simulink subsystem "vehicle_sim"  (R2025b)
settings: Solver=VariableStepAuto  StartTime=0.0  StopTime=10.0  RelTol=1e-3
libraries: vehdynlibsteering x1, autolibshared x1
settings Model: Creator=jessi  LastModifiedBy=jessi

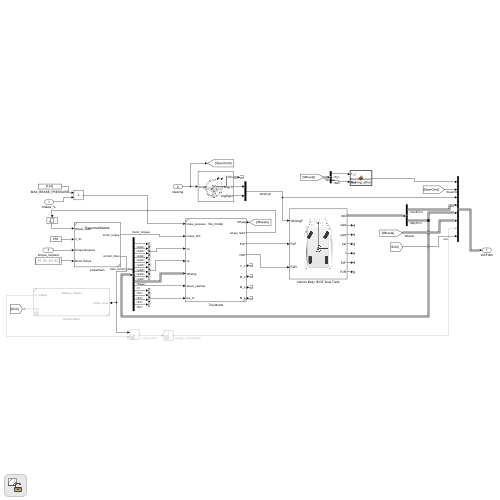
[thumbnail: Simulink's stored preview of the top-level diagram]
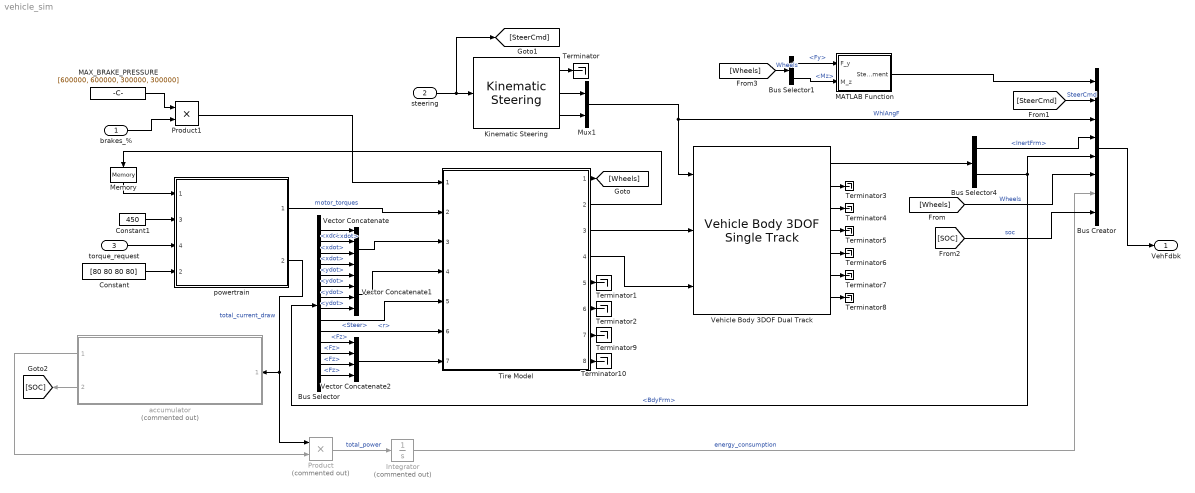
== system vehicle_sim ==
  brakes_% : Inport  PortDimensions=1
  steering : Inport  Port=2
  torque_request : Inport  Port=3  Unit=N*m  PortDimensions=4
  Bus Creator : BusCreator  Inputs=8
  Bus Selector : BusSelector  OutputSignals=FrntAxl.Lft.Vel.xdot,FrntAxl.Rght.Vel.xdot,RearAxl.Lft.Vel.xdot,RearAxl.Rght.Vel.xdot,FrntAxl.Lft.Vel.ydot,FrntAxl.Rght.Vel.ydot,RearAxl.Lft.Vel.ydot,RearAxl.Rght.Vel.ydot,FrntAxl.Steer,Cg.AngVel.r,Forces.Tires.FrntTires.Lft.Fz,Forces.Tires.FrntTires.Rght.Fz,Forces.Tires.RearTires.Lft.Fz,Forces.Tires.RearTires.Rght.Fz
  Bus Selector1 : BusSelector  OutputSignals=Fy,Mz
  Bus Selector4 : BusSelector  OutputSignals=InertFrm,BdyFrm
  Constant : Constant  Value=[80 80 80 80]
  Constant1 : Constant  Value=450
  Integrator : Integrator  Commented=on
  Kinematic Steering : vehdynlibsteering/Kinematic Steering  StrgType=Ackerman  StrgRatioType=Constant  Loc=Front  NrmlFctr=1  TrckWdth=1.1  WhlBase=1.550  Db=0  StrgRng=3*pi  StrgAngBpts="[-6.2832   -5.0265   -3.7699   -2.5133   -1.2566         0    1.2566    2.5133    3.7699    5.0265    6.2832]"  StrgRatioTbl=|  StrgRatio=10  PctAckIn=off  PctAck=100  PctAckTbl=ones(1,11)*100  StrgArmLngth=0.1  RckCsLngth=0.5  TieRodLngth=0.248  D=0.2  PnnRadius=0.00085818  PnnRadiusTbl="[0.0055    0.0055    0.0056    0.0057    0.0058    0.0057    0.0057    0.0057    0.0056    0.0055    0.0055]"  RodLngth=0.1  ParaArmLngth=0.9  aMode=2
      | [13.5000   13.3750   13.2500   13.1250   13.0000   13.0000   13.0000   13.1250   13.2500   13.3750   13.5000
      | ]
  MATLAB Function : MATLAB Function  TreatAsAtomicUnit=on
  MAX_BRAKE_PRESSURE : Constant  Value=[600000, 600000, 300000, 300000]
  Memory : Memory
  Mux1 : Mux  Inputs=2
  Product : Product  Commented=on
  Product1 : Product
  Terminator{,1..10} (11 alike) : Terminator
  Tire Model : Subsystem  ReferencedSubsystem=tire_model
  Vector Concatenate : Concatenate  NumInputs=4
  Vector Concatenate1 : Concatenate  NumInputs=4
  Vector Concatenate2 : Concatenate  NumInputs=4
  Vehicle Body 3DOF Dual Track : autolibshared/Vehicle Body 3DOF Single Track  trackMode=Dual  inputMode=External forces  frontSteerMode=on  rearSteerMode=off  windMode=off  muMode=off  extFMode=off  extMMode=off  htchFMode=off  htchMMode=off  extXo=off  extpsio=off  extxdoto=off  extro=off  extYo=off  extTamb=off  extydoto=off  aMode=2  NF=2  NR=2  m=252  a=0.803  b=0.747  h=0.20  dh=1  hh=0.2  X_o=0  xdot_o=0.1  CalphaMode=off  sigmaMode=on  d=0  hl=0  w=[0.775, 0.775]  Cy_f=12e3  Cy_r=11e3  sigma_f=.1  sigma_r=.1  alpha_f_brk=[-.1 .1]  Cy_f_data=[-9e3 9e3]  alpha_r_brk=[-.1 .1]  Cy_r_data=[-9e3 9e3]  Y_o=0  ydot_o=0  Izz=400  psi_o=0  r_o=0  Af=0.94  Cd=1.08  Cl=1.52  Cpm=.1  beta_w=[0 0.01:0.01:0.3]  Cs=[0:0.03:0.9]  Cym=[0 1e-6:0.01:0.3]  Pabs=101325  Tair=303  g=9.81  mu=1  xdot_tol=.01  Fznom=1961  Fxtire_sat=7e4  Fytire_sat=7e4  longOff=0  latOff=0  vertOff=0  wrapAng=off
      settings: LibrarySourceBlock=vehdynlibeom/Vehicle Body 3DOF Dual Track
  accumulator : Subsystem  Commented=on  ReferencedSubsystem=battery_model
      settings: PermitHierarchicalResolution=None
  powertrain : Subsystem  ReferencedSubsystem=PowertrainMatlab
      settings: PortSchema="{\"entries\":[{\"content\":{\"sides\":[{\"content\":{\"connectorIds\":[\"In1\",\"In3\",\"In4\",\"In2\"]},\"type\":\"ConnectorPlacement.EquallySpacedRectSide\",\"uuid\":\"bcaef28c-3728-4a2f-bdf4-b5e563d052c4\"},{\"content\":{\"connectorIds\":[\"Out1\",\"Out2\"],\"side\":\"RIGHT\"},\"type\":\"ConnectorPlacement.EquallySpacedRectSide\",\"uuid\":\"28426850-3a4f-491f-93a4-dadf03d879c7\"},{\"content\":{\"side\":\"TOP\"},\"type\":\"ConnectorPlacement.EquallySpacedRectSide\",\"uuid\":\"e3e154eb-71d0-41ee-9d2f-ecd68212e3aa\"}]},\"type\":\"ConnectorPlacement.EquallySpacedConnector\",\"uuid\":\"36c75ed7-43f2-403e-a237-5cc8486f527e\"}],\"packageUris\":[\"http://schema.mathworks.com/mf0/Connector/R2020b\"],\"version\":\"1.0\"}"
  VehFdbk : Outport
  wires:
  Bus Creator/1 -> VehFdbk/1
  Memory/1 -> powertrain/1
  Tire Model/8 -> Terminator10/1
  Tire Model/7 -> Terminator9/1
  Tire Model/6 -> Terminator2/1
  Tire Model/5 -> Terminator1/1
  brakes_%/1 -> Product1/2
  Bus Selector/3 -> Vector Concatenate/3  "<xdot>"
  Constant/1 -> powertrain/2
  Mux1/1 -> Vehicle Body 3DOF Dual Track/1, Bus Creator/3  "WhlAngF"
  Vehicle Body 3DOF Dual Track/5 -> Terminator6/1
  Bus Selector4/2 -> Bus Selector/1, Bus Creator/5  "<BdyFrm>"
  Bus Selector/7 -> Vector Concatenate1/3  "<ydot>"
  Bus Selector/13 -> Vector Concatenate2/3  "<Fz>"
  Bus Selector/11 -> Vector Concatenate2/1  "<Fz>"
  Bus Selector/5 -> Vector Concatenate1/1  "<ydot>"
  Vehicle Body 3DOF Dual Track/6 -> Terminator7/1
  Product/1 -> Integrator/1  "total_power"
  Bus Selector/1 -> Vector Concatenate/1  "<xdot>"
  Vehicle Body 3DOF Dual Track/3 -> Terminator4/1
  Bus Selector/6 -> Vector Concatenate1/2  "<ydot>"
  Kinematic Steering/1 -> Terminator/1
  Bus Selector/4 -> Vector Concatenate/4  "<xdot>"
  Vehicle Body 3DOF Dual Track/4 -> Terminator5/1
  Bus Selector/8 -> Vector Concatenate1/4  "<ydot>"
  accumulator/1 -> Product/2
  Product1/1 -> Tire Model/1
  steering/1 -> Kinematic Steering/1, [SteerCmd]
  Vehicle Body 3DOF Dual Track/7 -> Terminator8/1
  Kinematic Steering/2 -> Mux1/1
  Tire Model/4 -> Vehicle Body 3DOF Dual Track/3
  Bus Selector/12 -> Vector Concatenate2/2  "<Fz>"
  Tire Model/2 -> Memory/1
  Bus Selector4/1 -> Bus Creator/4  "<InertFrm>"
  Vehicle Body 3DOF Dual Track/1 -> Bus Selector4/1
  Integrator/1 -> Bus Creator/7  "energy_consumption"
  Tire Model/1 -> [Wheels]
  [SteerCmd] -> Bus Creator/2  "SteerCmd"
  Bus Selector/2 -> Vector Concatenate/2  "<xdot>"
  MAX_BRAKE_PRESSURE/1 -> Product1/1
  Bus Selector/10 -> Tire Model/6  "<r>"
  Bus Selector/9 -> Tire Model/5  "<Steer>"
  Vehicle Body 3DOF Dual Track/2 -> Terminator3/1
  powertrain/2 -> accumulator/1, Product/1  "total_current_draw"
  [Wheels] -> Bus Creator/6  "Wheels"
  Vector Concatenate1/1 -> Tire Model/4
  Kinematic Steering/3 -> Mux1/2
  Bus Selector/14 -> Vector Concatenate2/4  "<Fz>"
  Tire Model/3 -> Vehicle Body 3DOF Dual Track/2
  powertrain/1 -> Tire Model/2  "motor_torques"
  Vector Concatenate/1 -> Tire Model/3
  Vector Concatenate2/1 -> Tire Model/7
  accumulator/2 -> [SOC]
  [SOC] -> Bus Creator/8  "soc"
  Constant1/1 -> powertrain/3
  [Wheels] -> Bus Selector1/1  "Wheels"
  Bus Selector1/1 -> MATLAB Function/1(F_y)  "<Fy>"
  Bus Selector1/2 -> MATLAB Function/2(M_z)  "<Mz>"
  MATLAB Function/1(SteeringMoment) -> Bus Creator/1
  torque_request/1 -> powertrain/4

== matlab function vehicle_sim/MATLAB Function ==
  data: F_y input; SteeringMoment output; M_z input
function SteeringMoment = steering_effort(F_y, M_z)
    steerArmLength = 0.10;  % moment arm from steering axis to tie rod pickup point
    MT = 0.095;  % Mechanical Trail
    gearradius = 0.01905;  % Calculated from KAZ website

    Mtotal = MT .* -F_y + 0.9 * M_z;
    tieforce = (Mtotal(1) + Mtotal(2)) / steerArmLength; % positive force is to the left
    SteeringMoment = (tieforce * gearradius);
end
